simulink model "RaspberryPIModel"  (R2014a)
settings: Solver=FixedStepDiscrete  StartTime=0.0  StopTime=inf  RelTol=1e-3
undefined symbols (not defined in the file): strel
libraries: embdlinuxlib x2, dspindex x2, visiontextngfix x1, visionstatistics x1, visionmorphops x1, visionanalysis x1, raspberrypi_drivers x1
settings Model: SimulationMode=external  ExtModeTrigDuration=100  Creator=mbelge  LastModifiedBy=pcox
settings DataIOCC: SignalLoggingSaveFormat=ModelDataLogs
settings OptimizationCC: ExpressionDepthLimit=2147483647  OptimizeModelRefInitCode=on  LifeSpan=1
settings DebuggingCC: UnderspecifiedInitializationDetection=Classic  SolverPrmCheckMsg=none  FcnCallInpInsideContextMsg=EnableAllAsWarning  StateNameClashWarn=warning
settings HardwareCC: ProdLargestAtomicInteger=Long  ProdLargestAtomicFloat=Double  ProdEndianess=LittleEndian  ProdHWDeviceType=ARM Compatible->ARM Cortex
settings RTWCC: SystemTargetFile=realtime.tlc  GenerateMakefile=off  TemplateMakefile=realtime.tmf  Description=Real-Time Toolbox  RTWVerbose=off  ProcessScript=realtime_make_rtw_hook
settings CodeAppCC: CustomSymbolStrType=$N$R$M  InternalIdentifier=Classic
settings STFCustomTargetCC: TargetLibSuffix=.a  GenerateSampleERTMain=on  ConcurrentExecutionCompliant=off  GeneratePreprocessorConditionals=Use local settings  ERTCustomFileBanners=on  SupportNonInlinedSFcns=off  SupportVariableSizeSignals=on  MATLABClassNameForMDSCustomization=Simulink.SoftwareTarget.ERTCustomization  GRTInterface=off  SystemTargetFile=realtime.tlc
settings ERTTargetCC: CombineOutputUpdateFcns=off  SupportContinuousTime=on  SupportVariableSizeSignals=on  ExtMode=on  ExtModeMexArgs='192.168.0.10' 0 17725  ERTSrcFileBannerTemplate=realtime_code_template.cgt  ERTHdrFileBannerTemplate=realtime_code_template.cgt  ERTDataSrcFileTemplate=realtime_code_template.cgt  ERTDataHdrFileTemplate=realtime_code_template.cgt  ERTCustomFileTemplate=realtime_file_process.tlc

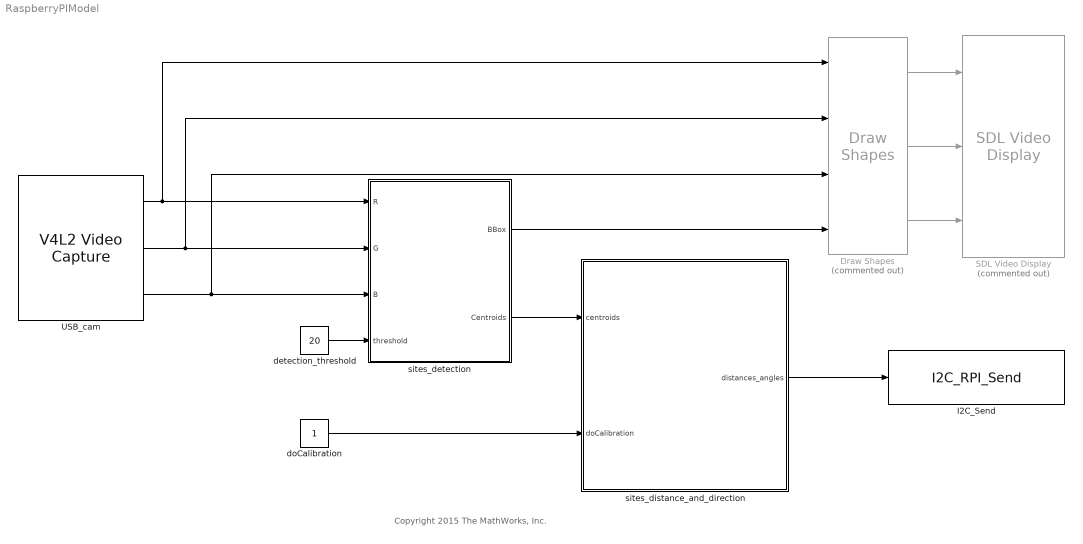
== system RaspberryPIModel ==
  note: Copyright 2015 The MathWorks, Inc.
  Draw Shapes : visiontextngfix/Draw Shapes  Commented=on  shape=Rectangles  fill=off  lineWidth=1  fillClrSource=Specify via dialog  display=User-specified value  intensity=200  color=[0 0 0]  opacity=0.6  viewport=Entire image  antialiasing=off  inType=Obsolete  imagePorts=Separate color signals  prodOutputMode=Binary point scaling  prodOutputWordLength=32  prodOutputFracLength=14  memoryMode=Specify word length  memoryWordLength=16  memoryFracLength=15  roundingMode=Floor  overflowMode=off
  I2C_Send : S-Function  InitFcn=try, set_param(gcb,'FunctionName','I2C_RPI_Send'), end  FunctionName=I2C_RPI_Send  SFunctionModules=I2C_RPI_Send_wrapper  EnableBusSupport=off  mask(S-Function Builder){}
      mask help: Simulink:masks:SFunctionBuilder_MD
      mask init:
      | val = [[.9  0.75 0.75 1 1 .9 .9 1]',[1 1 0.75 0.75 .9 .9 1 .9]'];try , sys = get_param(gcb,'SfunBuilderFcnName');if isempty(sys), sys = get_param(gcb,'FunctionName'); end,catch, sys = get_param(gcb,'FunctionName'); end
      settings: CopyFcn=set_param(gcbh,'LinkStatus','none')  PreSaveFcn=try, set_param(gcb,'FunctionName','I2C_RPI_Send'), end  OpenFcn=sfunctionwizard(gcbh)
      mask Display: plot(val(:,1),val(:,2)),disp(sys), port_label('input',1,'Send')
  SDL Video Display : embdlinuxlib/SDL Video Display  Commented=on  pixelFormat=RGB  pixelOrder=Planar  rowMajor=on  blockPlatform=Raspberry Pi
  USB_cam : embdlinuxlib/V4L2 Video Capture  m_devName='/dev/video0'  roi=[0, 0, 640, 480]  imSizeSelection=320x240  imSize=[640, 480]  pixelFormat=RGB  pixelOrder=Planar  sampleTime=1/10  simOutput=Colorbars  blockPlatform=Raspberry Pi
  detection_threshold : Constant  Value=20  OutDataTypeStr=single
  doCalibration : Constant  OutDataTypeStr=single
  sites_detection : Subsystem
  sites_distance_and_direction : Subsystem
  wires:
  USB_cam/3 -> Draw Shapes/3, sites_detection/3(B)
  USB_cam/2 -> Draw Shapes/2, sites_detection/2(G)
  USB_cam/1 -> Draw Shapes/1, sites_detection/1(R)
  Draw Shapes/3 -> SDL Video Display/3
  Draw Shapes/1 -> SDL Video Display/1
  Draw Shapes/2 -> SDL Video Display/2
  sites_detection/1(BBox) -> Draw Shapes/4
  detection_threshold/1 -> sites_detection/4(threshold)
  sites_detection/2(Centroids) -> sites_distance_and_direction/1(centroids)
  sites_distance_and_direction/1(distances_angles) -> I2C_Send/1
  doCalibration/1 -> sites_distance_and_direction/2(doCalibration)

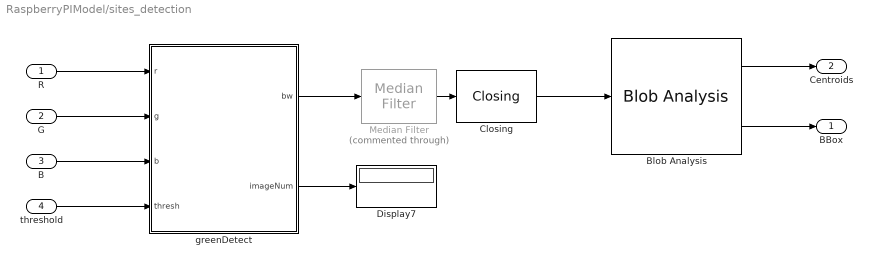
== system RaspberryPIModel/sites_detection ==
  R : Inport
  G : Inport  Port=2
  B : Inport  Port=3
  threshold : Inport  Port=4
  Blob Analysis : visionstatistics/Blob Analysis  Tag=vipblks_row_conv  area=off  centroid=on  bBox=on  majorAxis=off  minorAxis=off  angle=off  eccentricity=off  equivDiameterSq=off  extent=off  perimeter=off  maxBlobs=6  warnIfNumBlobsExceeded=off  isCount=off  useMinArea=on  minArea=25  useMaxArea=off  maxArea=intmax('uint32')  excludeBorderBlob=off  outDT=single  isOutVarDim=off  isFill=on  fillValues=-1  conn=8  isLabel=off  outputMode=Binary point scaling  outputWordLength=32  outputFracLength=16  firstCoeffMode=Binary point scaling  firstCoeffWordLength=16  firstCoeffFracLength=14  secondCoeffMode=Binary point scaling  secondCoeffWordLength=32  secondCoeffFracLength=16  accumMode=Binary point scaling  accumWordLength=32  accumFracLength=0  prodOutputMode=Binary point scaling  prodOutputWordLength=32  prodOutputFracLength=16  roundingMode=Floor  overflowMode=off
  Closing : visionmorphops/Closing  nhoodsrc=Specify via dialog  strel=strel('rectangle',[10 15])
  Display7 : Display
  Median Filter : visionanalysis/Median Filter  Commented=through  nghbood=[3 3]  outSize=Same as input port I  padType=Constant  padSrc=Specify via dialog  padVal=0  roundingMode=Floor  overflowMode=off
  greenDetect : MATLAB Function  TreatAsAtomicUnit=on
  BBox : Outport
  Centroids : Outport  Port=2
  wires:
  Closing/1 -> Blob Analysis/1
  Blob Analysis/2 -> BBox/1
  greenDetect/2(imageNum) -> Display7/1
  Median Filter/1 -> Closing/1
  greenDetect/1(bw) -> Median Filter/1
  threshold/1 -> greenDetect/4(thresh)
  R/1 -> greenDetect/1(r)
  B/1 -> greenDetect/3(b)
  G/1 -> greenDetect/2(g)
  Blob Analysis/1 -> Centroids/1

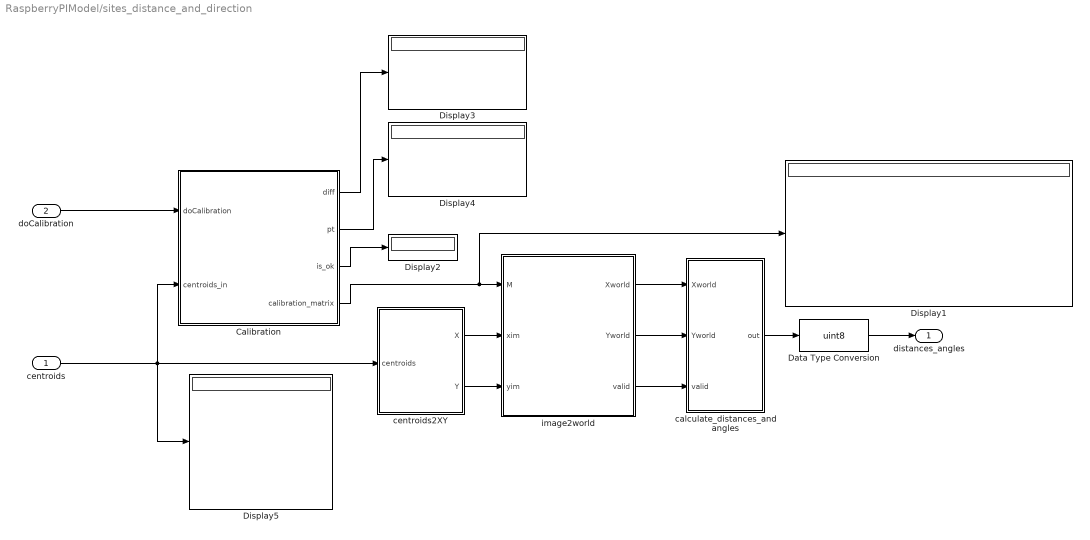
== system RaspberryPIModel/sites_distance_and_direction ==
  centroids : Inport
  doCalibration : Inport  Port=2
  Calibration : Stateflow chart  TreatAsAtomicUnit=on
  Data Type Conversion : DataTypeConversion  OutDataTypeStr=uint8
  Display{1..5} (5 alike) : Display
  calculate_distances_and angles : MATLAB Function  TreatAsAtomicUnit=on
  centroids2XY : Subsystem
  image2world : MATLAB Function  TreatAsAtomicUnit=on
  distances_angles : Outport
  wires:
  image2world/1(Xworld) -> calculate_distances_and angles/1(Xworld)
  image2world/2(Yworld) -> calculate_distances_and angles/2(Yworld)
  Data Type Conversion/1 -> distances_angles/1
  calculate_distances_and angles/1(out) -> Data Type Conversion/1
  image2world/3(valid) -> calculate_distances_and angles/3(valid)
  centroids/1 -> Display5/1, Calibration/2(centroids_in), centroids2XY/1(centroids)
  Calibration/4(calibration_matrix) -> Display1/1, image2world/1(M)
  Calibration/3(is_ok) -> Display2/1
  doCalibration/1 -> Calibration/1(doCalibration)
  centroids2XY/1(X) -> image2world/2(xim)
  centroids2XY/2(Y) -> image2world/3(yim)
  Calibration/1(diff) -> Display3/1
  Calibration/2(pt) -> Display4/1

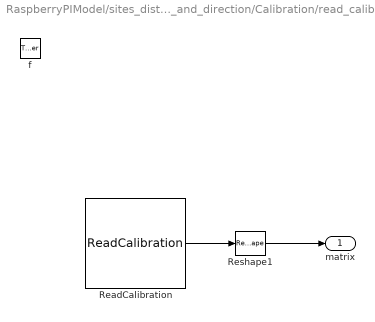
== system RaspberryPIModel/sites_distance_and_direction/Calibration/read_calibration ==
  f : TriggerPort  TriggerType=function-call
      settings: CopyFcn=Stateflow.SLINSF.SimulinkMan.removeBlockPreDeleteFcn  PreDeleteFcn=Stateflow.SLINSF.SimulinkMan.unsafePredeleteFcn
  ReadCalibration : S-Function  FunctionName=ReadCalibration  EnableBusSupport=off
  Reshape1 : Reshape  OutputDimensionality=Customize  OutputDimensions=[3,3]
  matrix : Outport  OutDataTypeStr=single  PortDimensions=[3 3]
  wires:
  ReadCalibration/1 -> Reshape1/1
  Reshape1/1 -> matrix/1

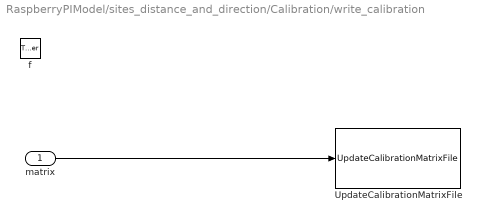
== system RaspberryPIModel/sites_distance_and_direction/Calibration/write_calibration ==
  matrix : Inport  OutDataTypeStr=single  PortDimensions=[3 3]
  f : TriggerPort  TriggerType=function-call
      settings: CopyFcn=Stateflow.SLINSF.SimulinkMan.removeBlockPreDeleteFcn  PreDeleteFcn=Stateflow.SLINSF.SimulinkMan.unsafePredeleteFcn
  UpdateCalibrationMatrixFile : raspberrypi_drivers/UpdateCalibrationMatrixFile
  wires:
  matrix/1 -> UpdateCalibrationMatrixFile/1

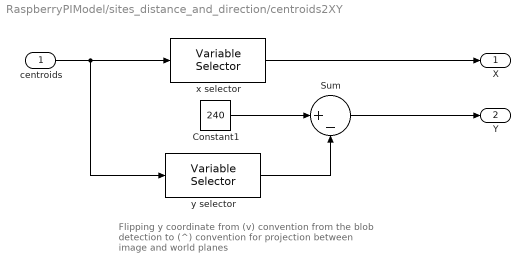
== system RaspberryPIModel/sites_distance_and_direction/centroids2XY ==
  note: Flipping y coordinate from (v) convention from
      | the blob detection to (^) convention for projection
      | between image and world planes
  centroids : Inport
  Constant1 : Constant  Value=240  OutDataTypeStr=single
  Sum : Sum  Inputs=|+-
  x selector : dspindex/Variable Selector  NumInputs=1  rowsOrCols=Columns  IdxMode=Fixed  Elements=2  ZerOneIdxMode=One-based  errmode=Generate Error  FillMode=on  FillValues=0
  y selector : dspindex/Variable Selector  NumInputs=1  rowsOrCols=Columns  IdxMode=Fixed  Elements=1  ZerOneIdxMode=One-based  errmode=Generate Error  FillMode=on  FillValues=0
  X : Outport
  Y : Outport  Port=2
  wires:
  x selector/1 -> X/1
  Constant1/1 -> Sum/1
  y selector/1 -> Sum/2
  Sum/1 -> Y/1
  centroids/1 -> y selector/1, x selector/1

== matlab function RaspberryPIModel/sites_detection/greenDetect ==
  data: r input; bw output; g input; b input; thresh input; imageNum output
function [bw, imageNum] = greenDetect(r, g, b, thresh)
%#codegen

persistent counter
if isempty(counter)
    counter = 1;
end
    

justGreen = single(g) - single(r)/2 - single(b)/2;
%justBlue = single(b) - single(r)/2 - single(g)/2;

bw = justGreen > thresh;
%bw = justBlue > thresh;

counter = counter + 1;
imageNum = counter;

== matlab function RaspberryPIModel/sites_distance_and_direction/image2world ==
  data: M input; Xworld output; xim input; yim input; Yworld output; valid output
function [Xworld, Yworld, valid] = image2world(M, xim, yim)
%#codegen

% Inputs: xim = [nx1] vector of x-coordinate in image plane
%         yim = [nx1] vector of y-coordinate in image plane
%         
%         For the image coordinates, origin is bottom left, convention:
%         x (>), y(^)
%
% Outputs: Xworld = [nx1] vector of x-coordinates in world plane
%          Yworld = [nx1] vector of y-coordinates in world plane
%          
%          For the world coordinates, robot at (X,Y) = (0,0)
%

% if size(xim, 2) > size(xim, 1)
%     xim = xim' ;
% end
% 
% if size(yim, 2) > size(yim, 1)
%     yim = yim' ;
% end
    
% [Xworld,Yworld] = transformPointsInverse(t_world2im, xim, yim) ;
% transformPointsInverse does not support codegen, but can get code from
% its class projective2d.

% M = inv( t_world2im );
u = M(1,1).*xim + M(2,1).*yim + M(3,1);
v = M(1,2).*xim + M(2,2).*yim + M(3,2);
w = M(1,3).*xim + M(2,3).*yim + M(3,3);

Xworld = u./w ;
Yworld = v./w ;

% limite the minimum Yworld to 0
%Yworld = max([Yworld, zeros(size(Yworld))],[],2) ;

valid = ~(xim == -1);

== matlab function RaspberryPIModel/sites_distance_and_direction/calculate_distances_and angles ==
  data: Xworld input; out output; Yworld input; valid input
function out  = fcn(Xworld, Yworld, valid)
%#codegen

angles = atan2d(Yworld , Xworld);
distances = sqrt(Xworld.^2 + Yworld.^2); % already in cm

angles = angles .* valid;
distances = distances .* valid;
out = [ distances', angles'];

== stateflow chart RaspberryPIModel/sites_distance_and_direction/Calibration ==
  state Calibration
    entry,during:
    [matrix,is_ok,pt,diff] = calibrate_camera(centroids_in);
  state Run
  state WriteCalibration
    entry:
    write_calibration(matrix);
  state matrix = read_calibration [function]
  state write_calibration(matrix) [function]
  (default) -> Run : {
      | calibration_matrix = read_calibration();
      | }
  Run -> Calibration : [doCalibration == 1]
  Calibration -> Run [order 2]
  (junction 10) -> Run : {
      | calibration_matrix = read_calibration();
      | }
  Calibration -> WriteCalibration [order 1] : [is_ok]
  WriteCalibration -> (junction 10)
  data: matrixProj function_output; centroids function_input; calibrated function_output; imagePoints function_output; difference function_output; matrix function_output single size=[3 3]; matrix function_input single size=[3 3]; diff output size=[4 2]; pt output size=[4 2]; is_ok output; doCalibration input; centroids_in input single size=[6 2]; calibration_matrix output single size=[3 3]; matrix local single size=[3 3]
  function [matrixProj,calibrated,imagePoints,difference] = calibrate_camera(centroids):
    | function [matrixProj,calibrated,imagePoints,difference] = calibrate_camera(centroids)
    | 
    | %#codegen
    | centroids = single(centroids);
    | % matrixProj = single( [-0.0101    0.0008    0.0000;
    | %                       -0.0002    0.0015    0.0005;
    | %                        1.7075   -3.4207   -0.1261] );
    | 
    | 
    | 
    | matrixProj = single( zeros(3,3) );
    | difference = single( zeros(4,2) );
    | calibrated = false;
    | 
    | 
    | % image points, pixel coordinates, assuming resolution of the camera =
    | % [240x320]
    | % (>) x (^) y
    | numPointsToUse = 4;
    | numrows = single(240) ;
    | yi = numrows - centroids(1:numPointsToUse, 1);  % from (v) to (^)
    | xi = centroids(1:numPointsToUse, 2); % (>)
    | 
    | % match the points to the 4 in the world
    | topPtsInds = yi > mean(yi) ;
    | bottomPtsInds = ~topPtsInds;
    | leftPtsInds = xi < mean(xi) ;
    | rightPtsInds = ~leftPtsInds ;
    | 
    | imagePoints = [xi(topPtsInds & leftPtsInds), yi(topPtsInds & leftPtsInds) ;             % top left
    |     xi(topPtsInds & rightPtsInds), yi(topPtsInds & rightPtsInds) ;           % top right
    |     xi(bottomPtsInds & leftPtsInds), yi(bottomPtsInds & leftPtsInds) ;       % bottom left
    |     xi( bottomPtsInds & rightPtsInds), yi(bottomPtsInds & rightPtsInds)];    % bottom right
    | 
    | % Do we have 4 and only 4 points? are they in the expected location?
    | imagePointsGT = [104 177;210 177;51 104;261 104]; % Ground Truth [4x2]
    | tolerance = 20;  % in pixels
    | 
    | difference(:) = abs(imagePoints - imagePointsGT);
    | wrongPtsDetected = sum(sum(difference > tolerance)) > 0;
    | 
    | if ~wrongPtsDetected
    |     % world points (for four points on corners of A3 paper)
    |     %     1      2
    |     %   3          4
    |     % + change of origin
    |     Xw = [0,    0.297,  0,  0.297  ] - 0.297/2; % (>)
    |     Yw = [0.42, 0.42,   0,  0] + 0.42; % (^)
    |     worldPoints = [Xw', Yw'] * 100; % in cm
    |     
    |     [worldPoints,normMatrix_world] = myNormalizeControlPoints(worldPoints);
    |     [imagePoints,normMatrix_image] = myNormalizeControlPoints(imagePoints);
    |     
    |     minRequiredNonCollinearPairs = 4;
    |     M = size(imagePoints,1);
    |     x = imagePoints(:,1);
    |     y = imagePoints(:,2);
    |     vec_1 = ones(M,1);
    |     vec_0 = zeros(M,1);
    |     u = worldPoints(:,1);
    |     v = worldPoints(:,2);
    |     
    |     U = [u; v];
    |     
    |     X = [x      y      vec_1  vec_0  vec_0  vec_0  -u.*x  -u.*y;
    |         vec_0  vec_0  vec_0  x      y      vec_1  -v.*x  -v.*y  ];
    |     
    |     Tvec = zeros(9,1,'single');
    |     % We know that X * Tvec = U
    |     if rank(X) >= 2*minRequiredNonCollinearPairs
    |         Tvec(1:8) = X \ U;
    |     else
    |         error('calib failed')
    |     end
    |     
    |     % We assumed I = 1;
    |     Tvec(9) = single(1);
    |     
    |     Tinv = reshape(Tvec,3,3);
    |     Tinv = normMatrix_image \ (Tinv * normMatrix_world);
    |     
    |     T = inv(Tinv);
    |     T = T ./ T(3,3);
    |     matrixProj = single( inv( T ) ); % image to world projection
    |     calibrated = true;
    | end
